simulink model "SixDoFRocketDynamics"  (R2022b)
settings: Solver=VariableStepAuto  StartTime=0.0  StopTime=30  RelTol=1e-3
undefined symbols (not defined in the file): Earth, WGS84
libraries: simulink x1, aerolibwind2 x1, aerolibtransform2 x1, aerolibatmos2 x1, aerolibasang x1, shared6dof x1
settings Model: Creator=nikil  LastModifiedBy=nikil

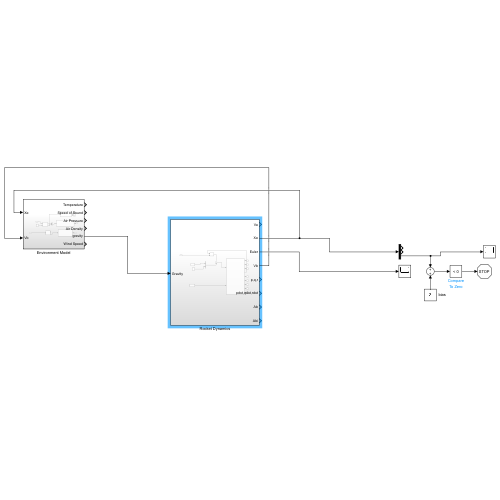
[thumbnail: Simulink's stored preview of the top-level diagram]
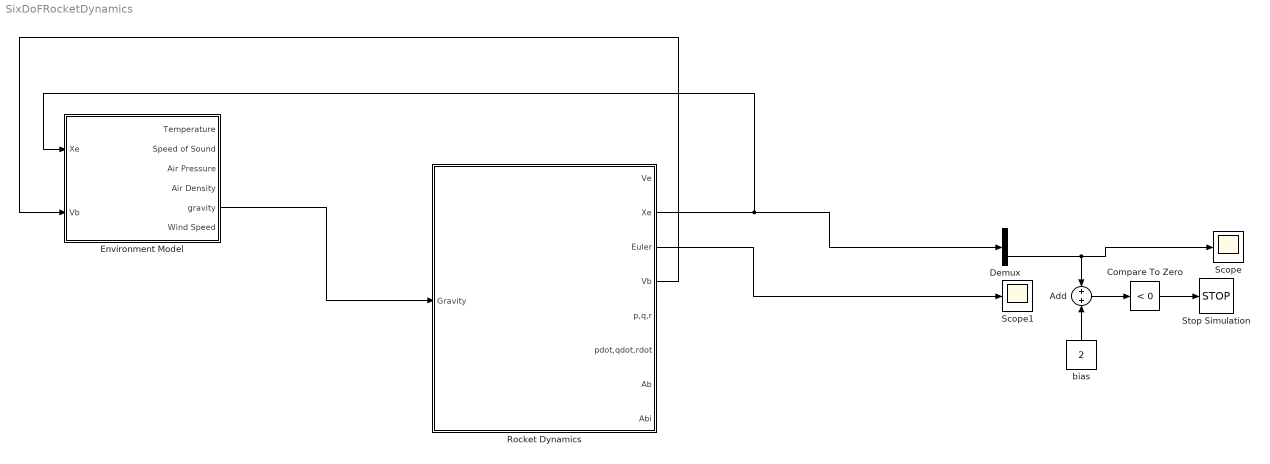
== system SixDoFRocketDynamics ==
  Add : Sum
  Compare To Zero : simulink/Logic and Bit Operations/Compare To Zero  relop=<  OutDataTypeStr=boolean
  Demux : Demux  Outputs=3
  Environment Model : Subsystem
  Rocket Dynamics : Subsystem
  Scope : Scope
  Scope1 : Scope
  Stop Simulation : Stop
  bias : Constant  Value=2
  wires:
  Demux/3 -> Add/1, Scope/1
  Add/1 -> Compare To Zero/1
  Compare To Zero/1 -> Stop Simulation/1
  bias/1 -> Add/2
  Rocket Dynamics/2(Xe) -> Environment Model/1(Xe), Demux/1
  Rocket Dynamics/4(Vb) -> Environment Model/2(Vb)
  Rocket Dynamics/3(Euler) -> Scope1/1
  Environment Model/5(gravity) -> Rocket Dynamics/1(Gravity)

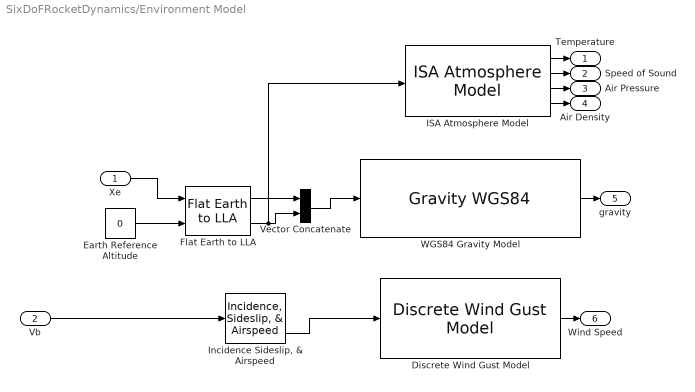
== system SixDoFRocketDynamics/Environment Model ==
  Xe : Inport
  Vb : Inport  Port=2
  Discrete Wind Gust Model : aerolibwind2/Discrete Wind Gust Model  units=Metric (MKS)  Gx=on  Gy=on  Gz=on  t_0=5  d_m=[120 120 80]  v_m=[3.5 3.5 3.0]
  Earth Reference Altitude : Constant  Value=0
  Flat Earth to LLA : aerolibtransform2/Flat Earth to LLA  units=Metric (MKS)  ptype=Earth (WGS84)  F=1/298.257223563  R=6378137  refPosPort=off  LL0=[0 10]  psi=0
  ISA Atmosphere Model : aerolibatmos2/ISA Atmosphere Model  custom=off  g=9.80665  gamma=1.4  R=287.0531  L=0.0065  h_trop=11000  h_strat=20000  rho0=1.225  P0=101325  T0=288.15  h0=0
  "Incidence Sideslip, & Airspeed" : aerolibasang/Incidence, Sideslip, & Airspeed
  Vector Concatenate : Concatenate
  "WGS84 Gravity Model  " : GravityWGS84
  Temperature : Outport
  Speed of Sound : Outport  Port=2
  Air Pressure : Outport  Port=3
  Air Density : Outport  Port=4
  gravity : Outport  Port=5
  Wind Speed : Outport  Port=6
  wires:
  "WGS84 Gravity Model  "/1 -> gravity/1
  Discrete Wind Gust Model/1 -> Wind Speed/1
  ISA Atmosphere Model/2 -> Speed of Sound/1
  ISA Atmosphere Model/3 -> Air Pressure/1
  ISA Atmosphere Model/1 -> Temperature/1
  ISA Atmosphere Model/4 -> Air Density/1
  Xe/1 -> Flat Earth to LLA/1
  Flat Earth to LLA/1 -> Vector Concatenate/1
  Flat Earth to LLA/2 -> ISA Atmosphere Model/1, Vector Concatenate/2
  Vector Concatenate/1 -> "WGS84 Gravity Model  "/1
  Earth Reference Altitude/1 -> Flat Earth to LLA/2
  Vb/1 -> "Incidence Sideslip, & Airspeed"/1
  "Incidence Sideslip, & Airspeed"/3 -> Discrete Wind Gust Model/1

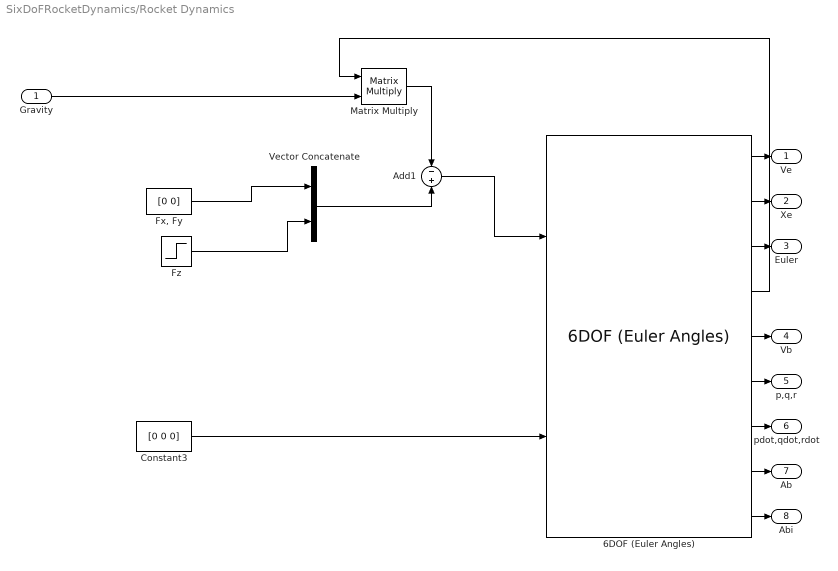
== system SixDoFRocketDynamics/Rocket Dynamics ==
  Gravity : Inport
  6DOF (Euler Angles) : shared6dof/6DOF (Euler Angles)  units=Metric (MKS)  mtype=Fixed  rep=Euler Angles  xme_0=[0 0 0]  Vm_0=[0 0 0]  eul_0=[0 0 0]  pm_0=[0 0 0]  mass_0=1.0  mass_e=0.5  mass_f=2.0  inertia=eye(3)  inertia_e=eye(3)  inertia_f=2*eye(3)  k_quat=1.0  vre_flag=on  abi_flag=on  aMode=0  xme_statename=''  Vm_statename=''  eul_statename=''  quat_statename=''  pm_statename=''  mass_statename=''
  Add1 : Sum  Inputs=-+
  Constant3 : Constant  Value=[0 0 0]
  "Fx, Fy" : Constant  Value=[0 0]
  Fz : Step  Time=2  Before=50  After=0  SampleTime=0
  Matrix Multiply : Product  Multiplication=Matrix(*)
  Vector Concatenate : Concatenate
  Ve : Outport
  Xe : Outport  Port=2
  Euler : Outport  Port=3
  Vb : Outport  Port=4
  p,q,r : Outport  Port=5
  pdot,qdot,rdot : Outport  Port=6
  Ab : Outport  Port=7
  Abi : Outport  Port=8
  wires:
  6DOF (Euler Angles)/1 -> Ve/1
  Matrix Multiply/1 -> Add1/1
  Fz/1 -> Vector Concatenate/2
  6DOF (Euler Angles)/2 -> Xe/1
  Constant3/1 -> 6DOF (Euler Angles)/2
  6DOF (Euler Angles)/9 -> Abi/1
  "Fx, Fy"/1 -> Vector Concatenate/1
  6DOF (Euler Angles)/8 -> Ab/1
  Vector Concatenate/1 -> Add1/2
  Add1/1 -> 6DOF (Euler Angles)/1
  6DOF (Euler Angles)/4 -> Matrix Multiply/1
  6DOF (Euler Angles)/6 -> p,q,r/1
  6DOF (Euler Angles)/5 -> Vb/1
  6DOF (Euler Angles)/7 -> pdot,qdot,rdot/1
  6DOF (Euler Angles)/3 -> Euler/1
  Gravity/1 -> Matrix Multiply/2
